simulink model "simu_ss_lqr"  (R2015a)
settings: Solver=ode3  StartTime=0.0  StopTime=100  FixedStep=0.001  RelTol=1e-3
values from neighbouring files (symbols this model uses):
  A = -b/m    (= -0.5)    [cruise_control_lqr.m]
  B = 1/m    (= 0.01)    [cruise_control_lqr.m]
  C = 1    [cruise_control_lqr.m]
  D = 0    [cruise_control_lqr.m]
undefined symbols (not defined in the file or in its folder): K
settings Model: Creator=Xiaotian  LastModifiedBy=Xiaotian

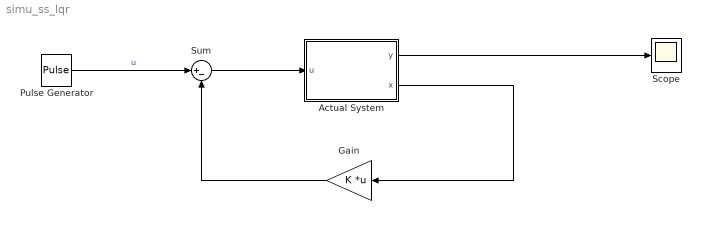
== system simu_ss_lqr ==
  Actual System : Subsystem  mask{A=A, B=B, C=C, D=D}
  Gain : Gain  Gain=K  Multiplication=Matrix(K*u)
  Pulse Generator : DiscretePulseGenerator  PulseType=Time based  Period=1000  PulseWidth=50
  Scope : Scope
  Sum : Sum  Inputs=|+-
  wires:
  Sum/1 -> Actual System/1(u)
  Pulse Generator/1 -> Sum/1  "u"
  Gain/1 -> Sum/2
  Actual System/1(y) -> Scope/1
  Actual System/2(x) -> Gain/1

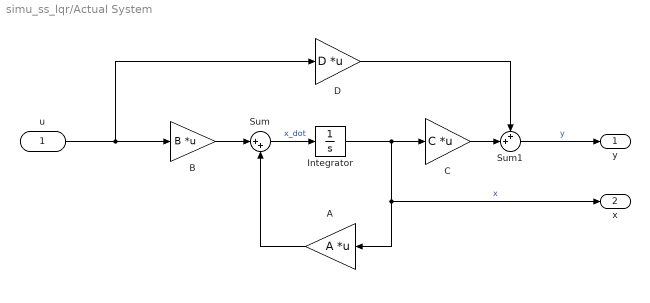
== system simu_ss_lqr/Actual System ==
  u : Inport
  A : Gain  Gain=A  Multiplication=Matrix(K*u)
  B : Gain  Gain=B  Multiplication=Matrix(K*u)
  C : Gain  Gain=C  Multiplication=Matrix(K*u)
  D : Gain  Gain=D  Multiplication=Matrix(K*u)
  Integrator : Integrator
  Sum : Sum  Inputs=|++
  Sum1 : Sum  Inputs=++|
  y : Outport
  x : Outport  Port=2
  wires:
  B/1 -> Sum/1
  Sum/1 -> Integrator/1  "x_dot"
  A/1 -> Sum/2
  u/1 -> D/1, B/1
  Sum1/1 -> y/1  "y"
  D/1 -> Sum1/1
  Integrator/1 -> x/1, A/1, C/1  "x"
  C/1 -> Sum1/2
